simulink model "Furnace"  (R2020a)
settings: Solver=ode15s  StartTime=0  StopTime=27000  FixedStep=0.1  MaxStep=20  MinStep=1e-13  RelTol=1e-08  AbsTol=1e-09
undefined symbols (not defined in the file): agnostic_lqe_params, cont_reg, disturbance_type, F_aI_pid, F_aII_pid, input_type, k, lqe_params, LQR_params, LQRAgnostic_params, MPC_type, MPCDiscrete_function_parameters, MPCDiscreteAgnostic_function_parameters, MPCDiscreteDiffIntegralAgnostic_function_parameters, original_LQR_params, output_type, reg, single_butter_ss
libraries: simulink x35, cstblocks x10, mpclib x3
(part 4 of 8)

== system Furnace/Deprecated, slow loop/Contineous Summer student feedback (Not finished)/Waste and Primary air ==
  "F_aI_reg_in " : Inport
  F_w_in_reg : Inport  Port=2
  Constant1 : Constant  Value=0
  Constant2 : Constant  Value=cont_reg.const_F_aI_dist
  Constant3 : Constant  Commented=on  Value=reg.const_T_aI
  Constant4 : Constant  Value=cont_reg.input_type_F_aI
  Constant5 : Constant  Commented=on  Value=reg.input_type_T_aI
  Constant6 : Constant  Value=cont_reg.input_type_F_w_in
  Constant7 : Constant  Value=cont_reg.input_type_F_aI
  Fiw_in1 : Constant  Commented=on  Value=k.w_w_in
  Flue gas fan : Subsystem
  From Workspace : FromWorkspace  Commented=on  VariableName=F_w_in
  Input selector : MATLAB Function  TreatAsAtomicUnit=on
  Input selector1 : MATLAB Function  Commented=on  TreatAsAtomicUnit=on
  Input selector2 : MATLAB Function  TreatAsAtomicUnit=on
  Input selector3 : MATLAB Function  TreatAsAtomicUnit=on
  PID Controller : simulink/Continuous/PID Controller  Controller=PI  Form=Parallel  TimeDomain=Continuous-time  UseExternalTs=off  SampleTime=1  IntegratorMethod=Forward Euler  FilterMethod=Forward Euler  ControllerParametersSource=internal  P=cont_reg.Kp_fan  I=cont_reg.Ki_fan  D=0  UseFilter=on  N=100  TunerSelectOption=Transfer Function Based (PID Tuner App)  InitialConditionSource=internal  InitialConditionForIntegrator=cont_reg.F_aI_fan_PID_int  InitialConditionForFilter=0  DifferentiatorICPrevScaledInput=0  ExternalReset=none  TrackingMode=off  Kt=1  LimitOutput=off  UpperSaturationLimit=inf  LowerSaturationLimit=-inf  LinearizeAsGain=on  AntiWindupMode=none  Kb=1  POutMin=[]  POutMax=[]  IOutMin=[]  IOutMax=[]  DOutMin=[]  DOutMax=[]  NOutMin=[]  NOutMax=[]  SumOutMin=[]  SumOutMax=[]  SaturationOutMin=[]  SaturationOutMax=[]  PParamMin=[]  PParamMax=[]  IParamMin=[]  IParamMax=[]  DParamMin=[]  DParamMax=[]  NParamMin=[]  NParamMax=[]  KbParamMin=[]  KbParamMax=[]  KtParamMin=[]  KtParamMax=[]  KbOutMin=[]  KbOutMax=[]  KtOutMin=[]  KtOutMax=[]  IntegratorOutMin=[]  IntegratorOutMax=[]  FilterOutMin=[]  FilterOutMax=[]  SumI1OutMin=[]  SumI1OutMax=[]  SumI2OutMin=[]  SumI2OutMax=[]  SumI3OutMin=[]  SumI3OutMax=[]  SumI4OutMin=[]  SumI4OutMax=[]  SumDOutMin=[]  SumDOutMax=[]  DifferentiatorOutMin=[]  DifferentiatorOutMax=[]  FilterDiffOutCoefMin=[]  FilterDiffOutCoefMax=[]  ReciprocalOutMin=[]  ReciprocalOutMax=[]  SumDenOutMin=[]  SumDenOutMax=[]  SumNumOutMin=[]  SumNumOutMax=[]  DivideOutMin=[]  DivideOutMax=[]  UdiffTsProdOutMin=[]  UdiffTsProdOutMax=[]  NTsProdOutMin=[]  NTsProdOutMax=[]  UintegralTsProdOutMin=[]  UintegralTsProdOutMax=[]  UngainTsProdOutMin=[]  UngainTsProdOutMax=[]  IntegratorContinuousStateAttributes=''  IntegratorStateMustResolveToSignalObject=off  IntegratorRTWStateStorageClass=Auto  FilterContinuousStateAttributes=''  FilterStateMustResolveToSignalObject=off  FilterRTWStateStorageClass=Auto  ParallelPVariant=InternalParameters  IdealPVariant=Disabled  IVariant=InternalParameters  DVariant=Disabled  IntegratorVariant=Continuous  SatVariant=Disabled  AWVariant=Passthrough  PCopyVariant=Disabled  TRVariant=Disabled  FdbkBlocksVariant=Forward  IdealPFdbkVariant=Disabled  SatFdbkVariant=Disabled  DerivativeFilterVariant=Disabled  NVariant=Disabled  NCopyVariant=Disabled_SignalSpec  FilterICVariant=Disabled  IntegratorICVariant=InternalICs  ExternalResetVariant=Disabled  TRSumVariant=Passthrough  SumFdbkVariant=Disabled  SumVariant=Sum_PI  TsampFilterVariant=InternalTs  TsampNgainVariant=Passthrough  TsampIntegralVariant=Passthrough
  Product : Product  Commented=on
  Product1 : Product
  Square perturbation : SignalGenerator  WaveForm=square  Amplitude=cont_reg.F_w_pert_amp  Frequency=cont_reg.F_w_pert_freq
  Sum : Sum  Inputs=++|
  Sum1 : Sum  Inputs=|+-
  T_aI : FromWorkspace  Commented=on  VariableName=T_aI
  Terminator : Terminator
  Terminator1 : Terminator
  Tw_in : Constant  Commented=on  Value=k.T_amb
  const_F_aI : Constant  Value=cont_reg.const_F_aI
  const_F_w_in : Constant  Value=cont_reg.const_F_w_in
  Fi_w_out : Outport  VectorParamsAs1DForOutWhenUnconnected=off
  Fi_aI_out : Outport  Port=2  VectorParamsAs1DForOutWhenUnconnected=off
  Fi_aI_out1 : Outport  Port=3  VectorParamsAs1DForOutWhenUnconnected=off
  Fi_aI_out2 : Outport  Port=4  VectorParamsAs1DForOutWhenUnconnected=off
  wires:
  Flue gas fan/3(Power consumption) -> Terminator1/1
  Flue gas fan/2(Pressure difference) -> Terminator/1
  Product1/1 -> Input selector/3(controlled)
  Input selector3/1(signal) -> Sum1/1  "F_aI_out"
  Constant7/1 -> Input selector/4(input_type)
  Flue gas fan/1(Volume flow) -> Product1/1, Sum1/2
  Constant2/1 -> Product1/2, Input selector/2(experimental), Input selector/1(constant)
  Constant1/1 -> Input selector3/2(experimental)
  "F_aI_reg_in "/1 -> Input selector3/3(controlled)
  const_F_aI/1 -> Input selector3/1(constant)  "const_F_aI"
  Sum1/1 -> PID Controller/1
  PID Controller/1 -> Flue gas fan/1(PID signal)
  Square perturbation/1 -> Sum/1
  Sum/1 -> Product/1, Fi_w_out/1
  Input selector2/1(signal) -> Sum/2  "F_w_in"
  const_F_w_in/1 -> Input selector2/1(constant)  "const_F_w_in"
  F_w_in_reg/1 -> Input selector2/3(controlled)
  Constant6/1 -> Input selector2/4(input_type)
  Constant3/1 -> Input selector1/1(constant)
  T_aI/1 -> Input selector1/2(experimental)
  Constant5/1 -> Input selector1/4(input_type)
  Constant4/1 -> Input selector3/4(input_type)
  Input selector/1(signal) -> Fi_aI_out/1  "F_aI_out"
  From Workspace/1 -> Input selector2/2(experimental)
  Fiw_in1/1 -> Product/2
  Tw_in/1 -> Fi_aI_out1/1
  Input selector1/1(signal) -> Fi_aI_out2/1  "T_aI_out"

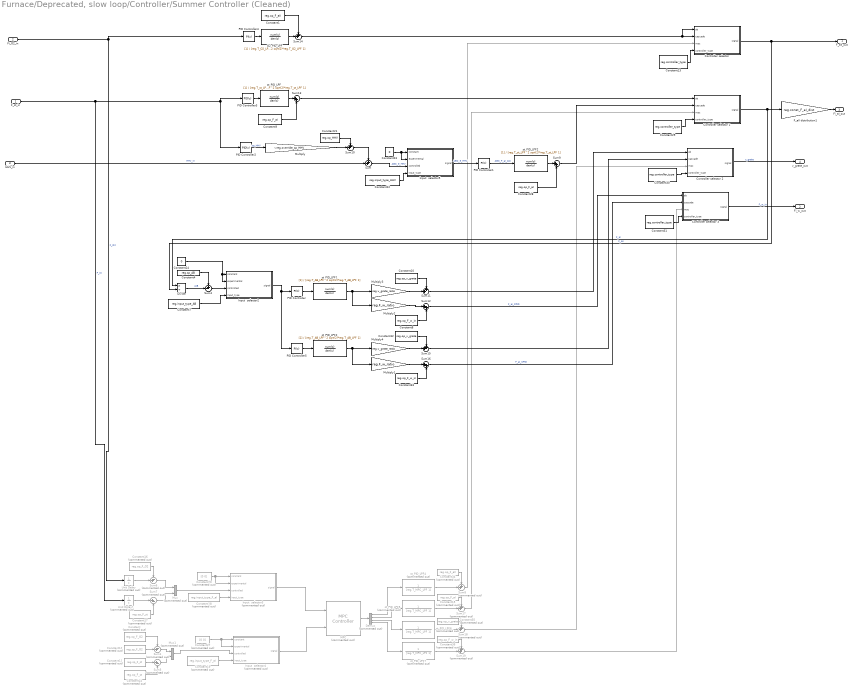
== system Furnace/Deprecated, slow loop/Controller/Summer Controller (Cleaned) ==
  F_st_in : Inport
  Fi_O2_in : Inport  Port=2
  HHV_in : Inport  Port=3
  Constant : Constant  Commented=on  Value=reg.op_F_O2
  Constant1 : Constant  Value=reg.op_F_aII
  Constant10 : Constant  Value=reg.op_v_grate
  Constant11 : Constant  Commented=on  Value=reg.sp_F_st
  Constant12 : Constant  Commented=on  Value=reg.sp_F_O2
  Constant{13,29..31} (4 alike) : Constant  Value=reg.controller_type
  Constant14 : Constant  Commented=on  Value=reg.op_F_st
  Constant15 : Constant  Commented=on  Value=reg.op_F_aI
  Constant16 : Constant  Commented=on  Value=reg.op_F_O2
  Constant17 : Constant  Commented=on  Value=reg.op_F_st
  Constant18 : Constant  Commented=on  Value=reg.input_type_F_aI
  Constant19 : Constant  Commented=on  Value=reg.input_type_F_aI
  Constant20 : Constant  Commented=on  Value=[0 0]
  Constant21 : Constant  Value=reg.op_HHV
  Constant22 : Constant  Value=reg.input_type_HHV
  Constant23 : Constant  Value=0
  Constant24 : Constant  Value=0
  Constant27 : Constant  Commented=on  Value=[0 0]
  Constant28 : Constant  Value=reg.op_F_aI
  Constant32 : Constant  Value=reg.op_v_grate
  Constant33 : Constant  Value=reg.op_F_w_in
  Constant34 : Constant  Commented=on  Value=reg.op_F_aII
  Constant35 : Constant  Commented=on  Value=reg.op_v_grate
  Constant36 : Constant  Commented=on  Value=reg.op_F_w_in
  Constant4 : Constant  Value=reg.sp_AB
  Constant7 : Constant  Value=reg.input_type_AB
  Constant8 : Constant  Value=reg.op_F_w_in
  Constant9 : Constant  Value=reg.op_F_aI
  "Controller selector " : MATLAB Function  TreatAsAtomicUnit=on
  Controller selector 1 : MATLAB Function  TreatAsAtomicUnit=on
  Controller selector 2 : MATLAB Function  TreatAsAtomicUnit=on
  Controller selector 3 : MATLAB Function  TreatAsAtomicUnit=on
  Demux : Demux  Commented=on
  Divide : Product  Inputs=*/  OutMin=[-100]  OutMax=[100]
  F_aII distribution1 : Gain  Gain=reg.const_F_aI_dist
  Input  selector2 : MATLAB Function  TreatAsAtomicUnit=on
  Input  selector3 : MATLAB Function  Commented=on  TreatAsAtomicUnit=on
  Input  selector4 : MATLAB Function  Commented=on  TreatAsAtomicUnit=on
  Input  selector5 : MATLAB Function  TreatAsAtomicUnit=on
  MPC : mpclib/MPC Controller  Commented=on  SCDEnableBlockLinearizationSpecification=on  mpcobj=lmpc  is_multiple=0  enable_value=0  return_u0=off  updateMPCinCallerWorkspace=on  md_inport=off  mv_inport=off  uref_inport=off  return_cost=off  return_mvseq=off  return_qpstatus=off  return_xseq=off  return_state=off  return_ovseq=off  state_inport=off  umin_inport=off  umax_inport=off  ymin_inport=off  ymax_inport=off  cc_inport=off  ywt_inport=off  uwt_inport=off  duwt_inport=off  rhoeps_inport=off  pm_inport=off  MaximumP=10  HorizonChoice=FixedHorizon  n_ts=20  n_p=50  n_mv=4  n_md=0  n_ud=0  n_mo=2  n_uo=0  BlockDataType=double  SampleTimeInherited=off  switch_inport=off
  Multiply : Gain  Gain=~reg.override_sp_HHV
  Multiply1 : Gain  Gain=reg.F_w_ratio
  Multiply2 : Gain  Gain=reg.F_w_ratio
  Multiply3 : Gain  Gain=reg.v_grate_ratio
  Multiply4 : Gain  Gain=reg.v_grate_ratio
  Mux : Mux  Commented=on  Inputs=2
  Mux1 : Mux  Commented=on  Inputs=2
  O2_PID_LPF : TransferFcn  Denominator=[reg.T_O2_LPF^2 sqrt(2)*reg.T_O2_LPF 1]
  PID Controller : simulink/Continuous/PID Controller  Controller=PI  Form=Parallel  TimeDomain=Discrete-time  UseExternalTs=off  SampleTime=1  IntegratorMethod=Forward Euler  FilterMethod=Forward Euler  ControllerParametersSource=internal  P=reg.Kp_AB  I=reg.Ki_AB  D=0  UseFilter=on  N=100  TunerSelectOption=Transfer Function Based (PID Tuner App)  InitialConditionSource=internal  InitialConditionForIntegrator=0  InitialConditionForFilter=0  DifferentiatorICPrevScaledInput=0  ExternalReset=none  TrackingMode=off  Kt=1  LimitOutput=off  UpperSaturationLimit=inf  LowerSaturationLimit=-inf  LinearizeAsGain=on  AntiWindupMode=none  Kb=1  POutMin=[]  POutMax=[]  IOutMin=[]  IOutMax=[]  DOutMin=[]  DOutMax=[]  NOutMin=[]  NOutMax=[]  SumOutMin=[]  SumOutMax=[]  SaturationOutMin=[]  SaturationOutMax=[]  PParamMin=[]  PParamMax=[]  IParamMin=[]  IParamMax=[]  DParamMin=[]  DParamMax=[]  NParamMin=[]  NParamMax=[]  KbParamMin=[]  KbParamMax=[]  KtParamMin=[]  KtParamMax=[]  KbOutMin=[]  KbOutMax=[]  KtOutMin=[]  KtOutMax=[]  IntegratorOutMin=[]  IntegratorOutMax=[]  FilterOutMin=[]  FilterOutMax=[]  SumI1OutMin=[]  SumI1OutMax=[]  SumI2OutMin=[]  SumI2OutMax=[]  SumI3OutMin=[]  SumI3OutMax=[]  SumI4OutMin=[]  SumI4OutMax=[]  SumDOutMin=[]  SumDOutMax=[]  DifferentiatorOutMin=[]  DifferentiatorOutMax=[]  FilterDiffOutCoefMin=[]  FilterDiffOutCoefMax=[]  ReciprocalOutMin=[]  ReciprocalOutMax=[]  SumDenOutMin=[]  SumDenOutMax=[]  SumNumOutMin=[]  SumNumOutMax=[]  DivideOutMin=[]  DivideOutMax=[]  UdiffTsProdOutMin=[]  UdiffTsProdOutMax=[]  NTsProdOutMin=[]  NTsProdOutMax=[]  UintegralTsProdOutMin=[]  UintegralTsProdOutMax=[]  UngainTsProdOutMin=[]  UngainTsProdOutMax=[]  IntegratorContinuousStateAttributes=''  IntegratorStateMustResolveToSignalObject=off  IntegratorRTWStateStorageClass=Auto  FilterContinuousStateAttributes=''  FilterStateMustResolveToSignalObject=off  FilterRTWStateStorageClass=Auto  ParallelPVariant=InternalParameters  IdealPVariant=Disabled  IVariant=InternalParameters  DVariant=Disabled  IntegratorVariant=Discrete  SatVariant=Disabled  AWVariant=Passthrough  PCopyVariant=Disabled  TRVariant=Disabled  FdbkBlocksVariant=Forward  IdealPFdbkVariant=Disabled  SatFdbkVariant=Disabled  DerivativeFilterVariant=Disabled  NVariant=Disabled  NCopyVariant=Disabled_SignalSpec  FilterICVariant=Disabled  IntegratorICVariant=InternalICs  ExternalResetVariant=Disabled  TRSumVariant=Passthrough  SumFdbkVariant=Disabled  SumVariant=Sum_PI  TsampFilterVariant=InternalTs  TsampNgainVariant=Passthrough  TsampIntegralVariant=Passthrough
  PID Controller1 : simulink/Continuous/PID Controller  Controller=PI  Form=Parallel  TimeDomain=Discrete-time  UseExternalTs=off  SampleTime=1  IntegratorMethod=Forward Euler  FilterMethod=Forward Euler  ControllerParametersSource=internal  P=reg.Kp_HHV  I=reg.Ki_HHV  D=0  UseFilter=on  N=100  TunerSelectOption=Transfer Function Based (PID Tuner App)  InitialConditionSource=internal  InitialConditionForIntegrator=0  InitialConditionForFilter=0  DifferentiatorICPrevScaledInput=0  ExternalReset=none  TrackingMode=off  Kt=1  LimitOutput=off  UpperSaturationLimit=inf  LowerSaturationLimit=-inf  LinearizeAsGain=on  AntiWindupMode=none  Kb=1  POutMin=[]  POutMax=[]  IOutMin=[]  IOutMax=[]  DOutMin=[]  DOutMax=[]  NOutMin=[]  NOutMax=[]  SumOutMin=[]  SumOutMax=[]  SaturationOutMin=[]  SaturationOutMax=[]  PParamMin=[]  PParamMax=[]  IParamMin=[]  IParamMax=[]  DParamMin=[]  DParamMax=[]  NParamMin=[]  NParamMax=[]  KbParamMin=[]  KbParamMax=[]  KtParamMin=[]  KtParamMax=[]  KbOutMin=[]  KbOutMax=[]  KtOutMin=[]  KtOutMax=[]  IntegratorOutMin=[]  IntegratorOutMax=[]  FilterOutMin=[]  FilterOutMax=[]  SumI1OutMin=[]  SumI1OutMax=[]  SumI2OutMin=[]  SumI2OutMax=[]  SumI3OutMin=[]  SumI3OutMax=[]  SumI4OutMin=[]  SumI4OutMax=[]  SumDOutMin=[]  SumDOutMax=[]  DifferentiatorOutMin=[]  DifferentiatorOutMax=[]  FilterDiffOutCoefMin=[]  FilterDiffOutCoefMax=[]  ReciprocalOutMin=[]  ReciprocalOutMax=[]  SumDenOutMin=[]  SumDenOutMax=[]  SumNumOutMin=[]  SumNumOutMax=[]  DivideOutMin=[]  DivideOutMax=[]  UdiffTsProdOutMin=[]  UdiffTsProdOutMax=[]  NTsProdOutMin=[]  NTsProdOutMax=[]  UintegralTsProdOutMin=[]  UintegralTsProdOutMax=[]  UngainTsProdOutMin=[]  UngainTsProdOutMax=[]  IntegratorContinuousStateAttributes=''  IntegratorStateMustResolveToSignalObject=off  IntegratorRTWStateStorageClass=Auto  FilterContinuousStateAttributes=''  FilterStateMustResolveToSignalObject=off  FilterRTWStateStorageClass=Auto  ParallelPVariant=InternalParameters  IdealPVariant=Disabled  IVariant=InternalParameters  DVariant=Disabled  IntegratorVariant=Discrete  SatVariant=Disabled  AWVariant=Passthrough  PCopyVariant=Disabled  TRVariant=Disabled  FdbkBlocksVariant=Forward  IdealPFdbkVariant=Disabled  SatFdbkVariant=Disabled  DerivativeFilterVariant=Disabled  NVariant=Disabled  NCopyVariant=Disabled_SignalSpec  FilterICVariant=Disabled  IntegratorICVariant=InternalICs  ExternalResetVariant=Disabled  TRSumVariant=Passthrough  SumFdbkVariant=Disabled  SumVariant=Sum_PI  TsampFilterVariant=InternalTs  TsampNgainVariant=Passthrough  TsampIntegralVariant=Passthrough
  PID Controller2 : simulink/Continuous/PID Controller  Controller=PID  Form=Parallel  TimeDomain=Discrete-time  UseExternalTs=off  SampleTime=1  IntegratorMethod=Forward Euler  FilterMethod=Forward Euler  ControllerParametersSource=internal  P=reg.Kp_st_HHV  I=reg.Ki_st_HHV  D=reg.Kd_st_HHV  UseFilter=on  N=100  TunerSelectOption=Transfer Function Based (PID Tuner App)  InitialConditionSource=internal  InitialConditionForIntegrator=0.001  InitialConditionForFilter=0  DifferentiatorICPrevScaledInput=0  ExternalReset=none  TrackingMode=off  Kt=1  LimitOutput=off  UpperSaturationLimit=inf  LowerSaturationLimit=1  LinearizeAsGain=on  AntiWindupMode=none  Kb=1  POutMin=[]  POutMax=[]  IOutMin=[]  IOutMax=[]  DOutMin=[]  DOutMax=[]  NOutMin=[]  NOutMax=[]  SumOutMin=[]  SumOutMax=[]  SaturationOutMin=[]  SaturationOutMax=[]  PParamMin=[]  PParamMax=[]  IParamMin=[]  IParamMax=[]  DParamMin=[]  DParamMax=[]  NParamMin=[]  NParamMax=[]  KbParamMin=[]  KbParamMax=[]  KtParamMin=[]  KtParamMax=[]  KbOutMin=[]  KbOutMax=[]  KtOutMin=[]  KtOutMax=[]  IntegratorOutMin=[]  IntegratorOutMax=[]  FilterOutMin=[]  FilterOutMax=[]  SumI1OutMin=[]  SumI1OutMax=[]  SumI2OutMin=[]  SumI2OutMax=[]  SumI3OutMin=[]  SumI3OutMax=[]  SumI4OutMin=[]  SumI4OutMax=[]  SumDOutMin=[]  SumDOutMax=[]  DifferentiatorOutMin=[]  DifferentiatorOutMax=[]  FilterDiffOutCoefMin=[]  FilterDiffOutCoefMax=[]  ReciprocalOutMin=[]  ReciprocalOutMax=[]  SumDenOutMin=[]  SumDenOutMax=[]  SumNumOutMin=[]  SumNumOutMax=[]  DivideOutMin=[]  DivideOutMax=[]  UdiffTsProdOutMin=[]  UdiffTsProdOutMax=[]  NTsProdOutMin=[]  NTsProdOutMax=[]  UintegralTsProdOutMin=[]  UintegralTsProdOutMax=[]  UngainTsProdOutMin=[]  UngainTsProdOutMax=[]  IntegratorContinuousStateAttributes='F_st'  IntegratorStateMustResolveToSignalObject=off  IntegratorRTWStateStorageClass=Auto  FilterContinuousStateAttributes=''  FilterStateMustResolveToSignalObject=off  FilterRTWStateStorageClass=Auto  ParallelPVariant=InternalParameters  IdealPVariant=Disabled  IVariant=InternalParameters  DVariant=InternalParameters  IntegratorVariant=Discrete  SatVariant=Disabled  AWVariant=Passthrough  PCopyVariant=Disabled  TRVariant=Disabled  FdbkBlocksVariant=Forward  IdealPFdbkVariant=Disabled  SatFdbkVariant=Disabled  DerivativeFilterVariant=ForwardEulerFilter  NVariant=InternalParameters  NCopyVariant=Disabled  FilterICVariant=InternalICsFilter  IntegratorICVariant=InternalICs  ExternalResetVariant=Disabled  TRSumVariant=Passthrough  SumFdbkVariant=Disabled  SumVariant=Sum_PID  TsampFilterVariant=InternalTs  TsampNgainVariant=Passthrough  TsampIntegralVariant=Passthrough
  PID Controller3 : simulink/Continuous/PID Controller  Controller=PID  Form=Parallel  TimeDomain=Discrete-time  UseExternalTs=off  SampleTime=1  IntegratorMethod=Forward Euler  FilterMethod=Forward Euler  ControllerParametersSource=internal  P=reg.Kp_st  I=reg.Ki_st  D=reg.Kd_st  UseFilter=on  N=100  TunerSelectOption=Transfer Function Based (PID Tuner App)  InitialConditionSource=internal  InitialConditionForIntegrator=0  InitialConditionForFilter=0  DifferentiatorICPrevScaledInput=0  ExternalReset=none  TrackingMode=off  Kt=1  LimitOutput=off  UpperSaturationLimit=inf  LowerSaturationLimit=1  LinearizeAsGain=on  AntiWindupMode=none  Kb=1  POutMin=[]  POutMax=[]  IOutMin=[]  IOutMax=[]  DOutMin=[]  DOutMax=[]  NOutMin=[]  NOutMax=[]  SumOutMin=[]  SumOutMax=[]  SaturationOutMin=[]  SaturationOutMax=[]  PParamMin=[]  PParamMax=[]  IParamMin=[]  IParamMax=[]  DParamMin=[]  DParamMax=[]  NParamMin=[]  NParamMax=[]  KbParamMin=[]  KbParamMax=[]  KtParamMin=[]  KtParamMax=[]  KbOutMin=[]  KbOutMax=[]  KtOutMin=[]  KtOutMax=[]  IntegratorOutMin=[]  IntegratorOutMax=[]  FilterOutMin=[]  FilterOutMax=[]  SumI1OutMin=[]  SumI1OutMax=[]  SumI2OutMin=[]  SumI2OutMax=[]  SumI3OutMin=[]  SumI3OutMax=[]  SumI4OutMin=[]  SumI4OutMax=[]  SumDOutMin=[]  SumDOutMax=[]  DifferentiatorOutMin=[]  DifferentiatorOutMax=[]  FilterDiffOutCoefMin=[]  FilterDiffOutCoefMax=[]  ReciprocalOutMin=[]  ReciprocalOutMax=[]  SumDenOutMin=[]  SumDenOutMax=[]  SumNumOutMin=[]  SumNumOutMax=[]  DivideOutMin=[]  DivideOutMax=[]  UdiffTsProdOutMin=[]  UdiffTsProdOutMax=[]  NTsProdOutMin=[]  NTsProdOutMax=[]  UintegralTsProdOutMin=[]  UintegralTsProdOutMax=[]  UngainTsProdOutMin=[]  UngainTsProdOutMax=[]  IntegratorContinuousStateAttributes='F_st'  IntegratorStateMustResolveToSignalObject=off  IntegratorRTWStateStorageClass=Auto  FilterContinuousStateAttributes=''  FilterStateMustResolveToSignalObject=off  FilterRTWStateStorageClass=Auto  ParallelPVariant=InternalParameters  IdealPVariant=Disabled  IVariant=InternalParameters  DVariant=InternalParameters  IntegratorVariant=Discrete  SatVariant=Disabled  AWVariant=Passthrough  PCopyVariant=Disabled  TRVariant=Disabled  FdbkBlocksVariant=Forward  IdealPFdbkVariant=Disabled  SatFdbkVariant=Disabled  DerivativeFilterVariant=ForwardEulerFilter  NVariant=InternalParameters  NCopyVariant=Disabled  FilterICVariant=InternalICsFilter  IntegratorICVariant=InternalICs  ExternalResetVariant=Disabled  TRSumVariant=Passthrough  SumFdbkVariant=Disabled  SumVariant=Sum_PID  TsampFilterVariant=InternalTs  TsampNgainVariant=Passthrough  TsampIntegralVariant=Passthrough
  PID Controller4 : simulink/Continuous/PID Controller  Controller=PI  Form=Parallel  TimeDomain=Discrete-time  UseExternalTs=off  SampleTime=1  IntegratorMethod=Forward Euler  FilterMethod=Forward Euler  ControllerParametersSource=internal  P=reg.Kp_O2  I=reg.Ki_O2  D=0  UseFilter=on  N=100  TunerSelectOption=Transfer Function Based (PID Tuner App)  InitialConditionSource=internal  InitialConditionForIntegrator=0.001  InitialConditionForFilter=0  DifferentiatorICPrevScaledInput=0  ExternalReset=none  TrackingMode=off  Kt=1  LimitOutput=off  UpperSaturationLimit=inf  LowerSaturationLimit=1  LinearizeAsGain=on  AntiWindupMode=none  Kb=1  POutMin=[]  POutMax=[]  IOutMin=[]  IOutMax=[]  DOutMin=[]  DOutMax=[]  NOutMin=[]  NOutMax=[]  SumOutMin=[]  SumOutMax=[]  SaturationOutMin=[]  SaturationOutMax=[]  PParamMin=[]  PParamMax=[]  IParamMin=[]  IParamMax=[]  DParamMin=[]  DParamMax=[]  NParamMin=[]  NParamMax=[]  KbParamMin=[]  KbParamMax=[]  KtParamMin=[]  KtParamMax=[]  KbOutMin=[]  KbOutMax=[]  KtOutMin=[]  KtOutMax=[]  IntegratorOutMin=[]  IntegratorOutMax=[]  FilterOutMin=[]  FilterOutMax=[]  SumI1OutMin=[]  SumI1OutMax=[]  SumI2OutMin=[]  SumI2OutMax=[]  SumI3OutMin=[]  SumI3OutMax=[]  SumI4OutMin=[]  SumI4OutMax=[]  SumDOutMin=[]  SumDOutMax=[]  DifferentiatorOutMin=[]  DifferentiatorOutMax=[]  FilterDiffOutCoefMin=[]  FilterDiffOutCoefMax=[]  ReciprocalOutMin=[]  ReciprocalOutMax=[]  SumDenOutMin=[]  SumDenOutMax=[]  SumNumOutMin=[]  SumNumOutMax=[]  DivideOutMin=[]  DivideOutMax=[]  UdiffTsProdOutMin=[]  UdiffTsProdOutMax=[]  NTsProdOutMin=[]  NTsProdOutMax=[]  UintegralTsProdOutMin=[]  UintegralTsProdOutMax=[]  UngainTsProdOutMin=[]  UngainTsProdOutMax=[]  IntegratorContinuousStateAttributes='F_st'  IntegratorStateMustResolveToSignalObject=off  IntegratorRTWStateStorageClass=Auto  FilterContinuousStateAttributes=''  FilterStateMustResolveToSignalObject=off  FilterRTWStateStorageClass=Auto  ParallelPVariant=InternalParameters  IdealPVariant=Disabled  IVariant=InternalParameters  DVariant=Disabled  IntegratorVariant=Discrete  SatVariant=Disabled  AWVariant=Passthrough  PCopyVariant=Disabled  TRVariant=Disabled  FdbkBlocksVariant=Forward  IdealPFdbkVariant=Disabled  SatFdbkVariant=Disabled  DerivativeFilterVariant=Disabled  NVariant=Disabled  NCopyVariant=Disabled_SignalSpec  FilterICVariant=Disabled  IntegratorICVariant=InternalICs  ExternalResetVariant=Disabled  TRSumVariant=Passthrough  SumFdbkVariant=Disabled  SumVariant=Sum_PI  TsampFilterVariant=InternalTs  TsampNgainVariant=Passthrough  TsampIntegralVariant=Passthrough
  PID Controller5 : simulink/Continuous/PID Controller  Controller=PI  Form=Parallel  TimeDomain=Discrete-time  UseExternalTs=off  SampleTime=1  IntegratorMethod=Forward Euler  FilterMethod=Forward Euler  ControllerParametersSource=internal  P=reg.Kp_AB_HHV  I=reg.Ki_AB_HHV  D=0  UseFilter=on  N=100  TunerSelectOption=Transfer Function Based (PID Tuner App)  InitialConditionSource=internal  InitialConditionForIntegrator=0  InitialConditionForFilter=0  DifferentiatorICPrevScaledInput=0  ExternalReset=none  TrackingMode=off  Kt=1  LimitOutput=off  UpperSaturationLimit=inf  LowerSaturationLimit=-inf  LinearizeAsGain=on  AntiWindupMode=none  Kb=1  POutMin=[]  POutMax=[]  IOutMin=[]  IOutMax=[]  DOutMin=[]  DOutMax=[]  NOutMin=[]  NOutMax=[]  SumOutMin=[]  SumOutMax=[]  SaturationOutMin=[]  SaturationOutMax=[]  PParamMin=[]  PParamMax=[]  IParamMin=[]  IParamMax=[]  DParamMin=[]  DParamMax=[]  NParamMin=[]  NParamMax=[]  KbParamMin=[]  KbParamMax=[]  KtParamMin=[]  KtParamMax=[]  KbOutMin=[]  KbOutMax=[]  KtOutMin=[]  KtOutMax=[]  IntegratorOutMin=[]  IntegratorOutMax=[]  FilterOutMin=[]  FilterOutMax=[]  SumI1OutMin=[]  SumI1OutMax=[]  SumI2OutMin=[]  SumI2OutMax=[]  SumI3OutMin=[]  SumI3OutMax=[]  SumI4OutMin=[]  SumI4OutMax=[]  SumDOutMin=[]  SumDOutMax=[]  DifferentiatorOutMin=[]  DifferentiatorOutMax=[]  FilterDiffOutCoefMin=[]  FilterDiffOutCoefMax=[]  ReciprocalOutMin=[]  ReciprocalOutMax=[]  SumDenOutMin=[]  SumDenOutMax=[]  SumNumOutMin=[]  SumNumOutMax=[]  DivideOutMin=[]  DivideOutMax=[]  UdiffTsProdOutMin=[]  UdiffTsProdOutMax=[]  NTsProdOutMin=[]  NTsProdOutMax=[]  UintegralTsProdOutMin=[]  UintegralTsProdOutMax=[]  UngainTsProdOutMin=[]  UngainTsProdOutMax=[]  IntegratorContinuousStateAttributes=''  IntegratorStateMustResolveToSignalObject=off  IntegratorRTWStateStorageClass=Auto  FilterContinuousStateAttributes=''  FilterStateMustResolveToSignalObject=off  FilterRTWStateStorageClass=Auto  ParallelPVariant=InternalParameters  IdealPVariant=Disabled  IVariant=InternalParameters  DVariant=Disabled  IntegratorVariant=Discrete  SatVariant=Disabled  AWVariant=Passthrough  PCopyVariant=Disabled  TRVariant=Disabled  FdbkBlocksVariant=Forward  IdealPFdbkVariant=Disabled  SatFdbkVariant=Disabled  DerivativeFilterVariant=Disabled  NVariant=Disabled  NCopyVariant=Disabled_SignalSpec  FilterICVariant=Disabled  IntegratorICVariant=InternalICs  ExternalResetVariant=Disabled  TRSumVariant=Passthrough  SumFdbkVariant=Disabled  SumVariant=Sum_PI  TsampFilterVariant=InternalTs  TsampNgainVariant=Passthrough  TsampIntegralVariant=Passthrough
  Sum{,10..11,14..15} (5 alike) : Sum  Inputs=++|
  Sum1 : Sum  Commented=on  Inputs=-+|
  Sum{9,12..13,16} (4 alike) : Sum  Inputs=|++
  Sum{8,17..19} (4 alike) : Sum  Commented=on  Inputs=++|
  Sum4 : Sum  Inputs=+-|
  Sum5 : Sum  Commented=on  Inputs=|+-
  Sum6 : Sum  Commented=on  Inputs=-+|
  Sum7 : Sum  Commented=on  Inputs=|+-
  Unit Delay : UnitDelay  Commented=on  HasFrameUpgradeWarning=on
  Unit Delay1 : UnitDelay  Commented=on  HasFrameUpgradeWarning=on
  st_PID_LPF : TransferFcn  Denominator=[reg.T_st_LPF^2 sqrt(2)*reg.T_st_LPF 1]
  st_PID_LPF1 : TransferFcn  Denominator=[reg.T_AB_LPF^2 sqrt(2)*reg.T_AB_LPF 1]
  st_PID_LPF2 : TransferFcn  Denominator=[reg.T_st_LPF^2 sqrt(2)*reg.T_st_LPF 1]
  st_PID_LPF3 : TransferFcn  Denominator=[reg.T_AB_LPF^2 sqrt(2)*reg.T_AB_LPF 1]
  st_PID_LPF{4..7} (4 alike) : TransferFcn  Commented=on  Denominator=[reg.T_MPC_LPF 1]
  F_aII_out : Outport  VectorParamsAs1DForOutWhenUnconnected=off
  Fi_w_out : Outport  Port=2  VectorParamsAs1DForOutWhenUnconnected=off
  Fi_aI_out : Outport  Port=3  VectorParamsAs1DForOutWhenUnconnected=off
  v_grate_out : Outport  Port=4  VectorParamsAs1DForOutWhenUnconnected=off
  wires:
  Multiply4/1 -> Sum15/2
  Multiply3/1 -> Sum11/2
  Sum19/1 -> Controller selector 3/3(mpc)
  Sum18/1 -> Controller selector 2/3(mpc)
  Sum8/1 -> "Controller selector "/3(mpc)
  Sum17/1 -> Controller selector 1/3(mpc)
  Constant36/1 -> Sum19/1
  Constant35/1 -> Sum18/1
  Constant15/1 -> Sum17/1
  Constant34/1 -> Sum8/1
  st_PID_LPF7/1 -> Sum19/2
  st_PID_LPF6/1 -> Sum18/2
  st_PID_LPF5/1 -> Sum17/2
  st_PID_LPF4/1 -> Sum8/2
  Unit Delay1/1 -> Sum7/1
  Unit Delay/1 -> Sum6/2
  Sum16/1 -> Controller selector 3/2(cascade)  "F_aI_CPID"
  Sum15/1 -> Controller selector 2/2(cascade)
  Multiply1/1 -> Sum16/1
  Constant32/1 -> Sum15/1
  Constant33/1 -> Sum16/2
  PID Controller5/1 -> st_PID_LPF3/1
  st_PID_LPF3/1 -> Multiply4/1, Multiply1/1
  Constant31/1 -> Controller selector 3/4(controller_type)
  Constant30/1 -> Controller selector 2/4(controller_type)
  Constant29/1 -> Controller selector 1/4(controller_type)
  Constant13/1 -> "Controller selector "/4(controller_type)
  Constant1/1 -> Sum14/1
  O2_PID_LPF/1 -> Sum14/2
  Constant9/1 -> Sum13/2
  Constant28/1 -> Sum9/2
  Sum6/1 -> Mux/1
  Sum1/1 -> Mux1/1
  st_PID_LPF2/1 -> Sum9/1
  Sum10/1 -> Sum/1
  Constant21/1 -> Sum10/1
  Multiply/1 -> Sum10/2
  PID Controller2/1 -> Multiply/1  "sp_HHV"
  Sum9/1 -> Controller selector 1/2(cascade)
  PID Controller1/1 -> st_PID_LPF2/1  "ABC_F_aI_out"
  Sum12/1 -> Controller selector 3/1(ab)  "F_aI_CPID"
  Constant27/1 -> Input  selector4/1(constant), Input  selector4/2(experimental)
  F_st_in/1 -> PID Controller3/1, PID Controller2/1, Unit Delay1/1  "F_st"
  Constant24/1 -> Input  selector2/1(constant), Input  selector2/2(experimental)
  Input  selector2/1(signal) -> PID Controller/1, PID Controller5/1
  Sum4/1 -> Input  selector2/3(controlled)
  Divide/1 -> Sum4/2  "A/B"
  Constant23/1 -> Input  selector5/1(constant), Input  selector5/2(experimental)
  Sum/1 -> Input  selector5/3(controlled)  "ABC_e_HHV"
  Constant22/1 -> Input  selector5/4(input_type)
  Input  selector5/1(signal) -> PID Controller1/1  "ABC_e_HHV"
  HHV_in/1 -> Sum/2  "HHV_in"
  Constant20/1 -> Input  selector3/1(constant), Input  selector3/2(experimental)
  Input  selector4/1(signal) -> MPC/2
  Mux1/1 -> Input  selector4/3(controlled)
  Constant19/1 -> Input  selector4/4(input_type)
  Constant18/1 -> Input  selector3/4(input_type)
  Mux/1 -> Input  selector3/3(controlled)
  Input  selector3/1(signal) -> MPC/1
  Constant17/1 -> Sum7/2
  Constant16/1 -> Sum6/1
  Sum7/1 -> Mux/2
  MPC/1 -> Demux/1
  Sum5/1 -> Mux1/2
  Constant14/1 -> Sum5/2
  Constant11/1 -> Sum5/1
  Constant/1 -> Sum1/1
  Constant12/1 -> Sum1/2
  Controller selector 3/1(signal) -> Fi_w_out/1  "F_w_in"
  Controller selector 2/1(signal) -> v_grate_out/1  "v_grate"
  Controller selector 1/1(signal) -> F_aII distribution1/1, Divide/1  "F_aI"
  "Controller selector "/1(signal) -> F_aII_out/1, Divide/2  "F_aII"
  Demux/4 -> st_PID_LPF7/1
  Demux/3 -> st_PID_LPF6/1
  Demux/2 -> st_PID_LPF5/1
  Demux/1 -> st_PID_LPF4/1
  st_PID_LPF1/1 -> Multiply3/1, Multiply2/1
  st_PID_LPF/1 -> Sum13/1
  Constant10/1 -> Sum11/1
  Multiply2/1 -> Sum12/1
  Sum11/1 -> Controller selector 2/1(ab)
  PID Controller/1 -> st_PID_LPF1/1
  Constant8/1 -> Sum12/2
  Sum13/1 -> Controller selector 1/1(ab)
  PID Controller3/1 -> st_PID_LPF/1
  Sum14/1 -> "Controller selector "/2(cascade), "Controller selector "/1(ab)
  PID Controller4/1 -> O2_PID_LPF/1
  Constant4/1 -> Sum4/1
  Constant7/1 -> Input  selector2/4(input_type)
  Fi_O2_in/1 -> PID Controller4/1, Unit Delay/1  "F_O2"
  F_aII distribution1/1 -> Fi_aI_out/1
